simulink model "CollisionSim"  (R2015a)
settings: Solver=ode45  StartTime=0.0  StopTime=70  FixedStep=0.001  RelTol=1e-3
values from neighbouring files (symbols this model uses):
  Destination_Obs = [1000,0]    [CD.m]
  K_eta = 1    [CD.m]    (also in PathFollowCompScript.m = 0.21)
  lambda_0 = atan2(lambda_vec_0(2),lambda_vec_0(1))    [CD.m]    (also in PathFollowCompScript.m)
  V_obs_max = 20    [CD.m]
undefined symbols (not defined in the file): Initial_Head_Obs, Initial_Heading, Initial_Pos_Obs, Initial_Position
libraries: simulink x4, aerolibtransform2 x1
settings Model: CovSFcnEnable=off  Creator=marinho  LastModifiedBy=marinho
settings DebuggingCC: UnderspecifiedInitializationDetection=Classic  MergeDetectMultiDrivingBlocksExec=none  SolverPrmCheckMsg=warning

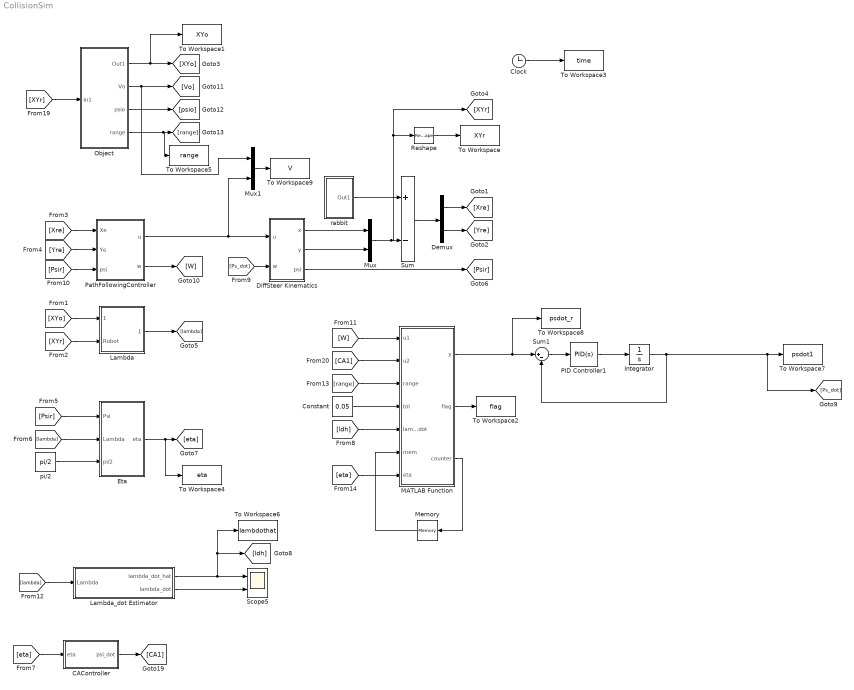
== system CollisionSim ==
  CAController : Subsystem
  Clock : Clock
  Constant : Constant  Value=0.05
  Demux : Demux  Outputs=2
  DiffSteer Kinematics : Subsystem  AncestorBlock=DiffSteer_model/DiffSteer Kinematics  mask{x0=[Initial_Position Initial_Heading], a=0.2, umax=32, wmax=5, dumax=inf, dwmax=inf}
      mask prompts: x0 "Initial pose [x, y, psi]"; a "Distance from traction wheels axis center to the point of interest [m]"; umax "Maximum linear velocity [m/s]"; wmax "Maximum angular velocity [rad/s]"; dumax "Maximum linear acceleration [m/s^2]"; dwmax "Maximum angular acceleration [rad/s^2]"
      mask help: Kinematics of the differential steered vehicle
      mask Help:
      | Kinematics of the differential steered vehicle (unicycle-like).
      | 
      | A differential steered (or differential wheeled) robot has two separately driven wheels placed on either side of its structure. Its orientation is changed by varying the relative velocities of its wheels.
      | In this model, robot position [x,y] is the position of the point of interest, which is located on a distance "a" from the center of the line that connects both traction wheels. If a = 0, this model is equal to the unicycle.
      | 
      | <b>Parameters:</b>
      | 
      | Initial pose: Vehicle initial position and orientation on absolute reference frame [x_0, y_0, psi_0]
      | Distance between traction wheels axis and point of interest (1x1): a [m]
      | Maximum Linear velocity (1x1):  Vehicle speed limit [m/s] (umax)
      | Maximum Angular velocity (1x1):  Vehicle turning velocity limit [rad/s] (wmax)
      | Maximum linear acceleration (1x1): Vehicle linear acceleration limit [m/s2] (dumax)
      | Maximum angular acceleration (1x1): Vehicle angular acceleration limit [rad/s2] (dwmax)
      | 
      | 
      | <b>Inputs:</b>
      | 
      | u (1x1): reference for linear velocity [m/s]
      | w (1x1): reference for angular velocity [rad/s]
      | 
      | <b>Outputs:</b>
      | 
      | x (1x1): x-coordinate in world frame [m]
      | y (1x1): y-coordinate in world frame [m]
      | psi (1x1): heading angle in world frame [rad]
      | 
      | <b>Notes:</b>
      | 
      | 1. If a = 0, this model is equal to the unicycle.
      | 
      | 2. This model does not take into account the robot dynamics. It considers that the actual robot velocity is exactly equal to the reference velocity (if it is bellow its limit).
      | 
      | For more information on the robot kinematics and dynamics, please refer to:
      | 
      | [1] MARTINS, F.N., CARELLI, R., SARCINELLI-FILHO, M. and BASTOS-FILHO, T.F.
      | Dynamic Modeling and Adaptive Dynamic Compensation for Unicycle-Like
      | Mobile Robots. 14th International Conference on Advanced Robotics -
      | ICAR 2009, Germany, June, 22-26, 2009.
      | 
      | [2] MARTINS, F.N., CELESTE, W.C., CARELLI, R., SARCINELLI-FILHO, M. and
      | BASTOS-FILHO, T.F. An Adaptive Dynamic Controller for Autonomous Mobile Robot
      | Trajectory Tracking. Control Engineering Practice, v. 16, p. 1354–1363, 2008.
      | doi: 10.1016/j.conengprac.2008.03.004
  Eta : Subsystem
  Integrator : Integrator  UpperSaturationLimit=0.5  LowerSaturationLimit=-0.5
  Lambda : Subsystem
  Lambda_dot Estimator : Subsystem
  MATLAB Function : MATLAB Function  TreatAsAtomicUnit=on
  Memory : Memory
  Mux : Mux  Inputs=2
  Mux1 : Mux  Inputs=2
  Object : Subsystem
  PID Controller1 : simulink/Continuous/PID Controller  Controller=PID  TimeDomain=Continuous-time  SampleTime=-1  IntegratorMethod=Forward Euler  FilterMethod=Forward Euler  Form=Parallel  UseFilter=on  ControllerParametersSource=internal  P=1  I=0  D=0.05  N=100  InitialConditionSource=internal  InitialConditionForIntegrator=0  InitialConditionForFilter=0  ExternalReset=none  LimitOutput=off  UpperSaturationLimit=0.1  LowerSaturationLimit=-0.1  LinearizeAsGain=on  AntiWindupMode=none  Kb=1  TrackingMode=off  Kt=1  PParamMin=[]  PParamMax=[]  IParamMin=[]  IParamMax=[]  DParamMin=[]  DParamMax=[]  NParamMin=[]  NParamMax=[]  KbParamMin=[]  KbParamMax=[]  KtParamMin=[]  KtParamMax=[]  POutMin=[]  POutMax=[]  IOutMin=[]  IOutMax=[]  DOutMin=[]  DOutMax=[]  NOutMin=[]  NOutMax=[]  KbOutMin=[]  KbOutMax=[]  KtOutMin=[]  KtOutMax=[]  IntegratorOutMin=[]  IntegratorOutMax=[]  FilterOutMin=[]  FilterOutMax=[]  SumOutMin=[]  SumOutMax=[]  SumI1OutMin=[]  SumI1OutMax=[]  SumI2OutMin=[]  SumI2OutMax=[]  SumI3OutMin=[]  SumI3OutMax=[]  SumDOutMin=[]  SumDOutMax=[]  SaturationOutMin=[]  SaturationOutMax=[]  IntegratorContinuousStateAttributes=''  IntegratorStateMustResolveToSignalObject=off  IntegratorRTWStateStorageClass=Auto  FilterContinuousStateAttributes=''  FilterStateMustResolveToSignalObject=off  FilterRTWStateStorageClass=Auto  DifferentiatorICPrevScaledInput=0  DifferentiatorOutMin=[]  DifferentiatorOutMax=[]
  PathFollowingController : Subsystem
  Reshape : Reshape
  Scope5 : Scope  NumInputPorts=2
      settings: YMin=-5~-5  YMax=5~5  SaveName=ScopeData10
  Sum : Sum  Inputs=+-
  Sum1 : Sum  Inputs=|+-
  To Workspace : ToWorkspace  VariableName=XYr  SampleTime=-1
  To Workspace1 : ToWorkspace  VariableName=XYo  SampleTime=-1
  To Workspace2 : ToWorkspace  VariableName=flag  SampleTime=-1
  To Workspace3 : ToWorkspace  VariableName=time  SampleTime=-1
  To Workspace4 : ToWorkspace  VariableName=eta  SampleTime=-1
  To Workspace5 : ToWorkspace  VariableName=range  SampleTime=-1
  To Workspace6 : ToWorkspace  VariableName=lambdothat  SampleTime=-1
  To Workspace7 : ToWorkspace  VariableName=psdot1  SampleTime=-1
  To Workspace8 : ToWorkspace  VariableName=psdot_r  SampleTime=-1
  To Workspace9 : ToWorkspace  VariableName=V  SampleTime=-1
  "pi/2 " : Constant  Value=pi/2  VectorParams1D=off  SampleTime=-1
  rabbit : Subsystem
  wires:
  DiffSteer Kinematics/1(x) -> Mux/1
  DiffSteer Kinematics/2(y) -> Mux/2
  Mux/1 -> Sum/2, [XYr], Reshape/1
  rabbit/1(Out1) -> Sum/1
  Sum/1 -> Demux/1
  Demux/2 -> [Yre]
  Demux/1 -> [Xre]
  Reshape/1 -> To Workspace/1
  DiffSteer Kinematics/3(psi) -> [Psir]
  [Xre] -> PathFollowingController/1(Xe)
  [Yre] -> PathFollowingController/2(Ye)
  [Psir] -> PathFollowingController/3(psi)
  PathFollowingController/1(u) -> Mux1/2, DiffSteer Kinematics/1(u)
  [W] -> MATLAB Function/1(u1)
  Clock/1 -> To Workspace3/1
  PathFollowingController/2(w) -> [W]
  [lambda] -> Lambda_dot Estimator/1(Lambda)
  Object/2(Vo) -> Mux1/1, [Vo]
  Object/3(psio) -> [psio]
  [XYr] -> Object/1(In1)
  MATLAB Function/2(flag) -> To Workspace2/1
  Lambda_dot Estimator/1(lambda_dot_hat) -> [ldh], To Workspace6/1, Scope5/1
  Lambda_dot Estimator/2(lambda_dot) -> Scope5/2
  Object/4(range) -> To Workspace5/1, [range]
  [range] -> MATLAB Function/3(range)
  MATLAB Function/3(counter) -> Memory/1
  Memory/1 -> MATLAB Function/6(mem)
  Constant/1 -> MATLAB Function/4(tol)
  [eta] -> MATLAB Function/7(eta)
  [Ps_dot] -> DiffSteer Kinematics/2(w)
  Object/1(Out1) -> To Workspace1/1, [XYo]
  [XYo] -> Lambda/1(Object)
  [XYr] -> Lambda/2(Robot)
  Lambda/1(Lambda) -> [lambda]
  Eta/1(eta) -> To Workspace4/1, [eta]
  [Psir] -> Eta/1(Psi)
  [lambda] -> Eta/2(Lambda)
  "pi/2 "/1 -> Eta/3(pi/2)
  [ldh] -> MATLAB Function/5(lambda_dot)
  [eta] -> CAController/1(eta)
  CAController/1(psi_dot) -> [CA1]
  Sum1/1 -> PID Controller1/1
  PID Controller1/1 -> Integrator/1
  MATLAB Function/1(y) -> To Workspace8/1, Sum1/1
  Integrator/1 -> [Ps_dot], To Workspace7/1, Sum1/2
  Mux1/1 -> To Workspace9/1
  [CA1] -> MATLAB Function/2(u2)

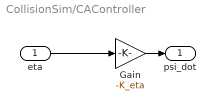
== system CollisionSim/CAController ==
  eta : Inport
  Gain : Gain  Gain=-K_eta
  psi_dot : Outport
  wires:
  Gain/1 -> psi_dot/1
  eta/1 -> Gain/1

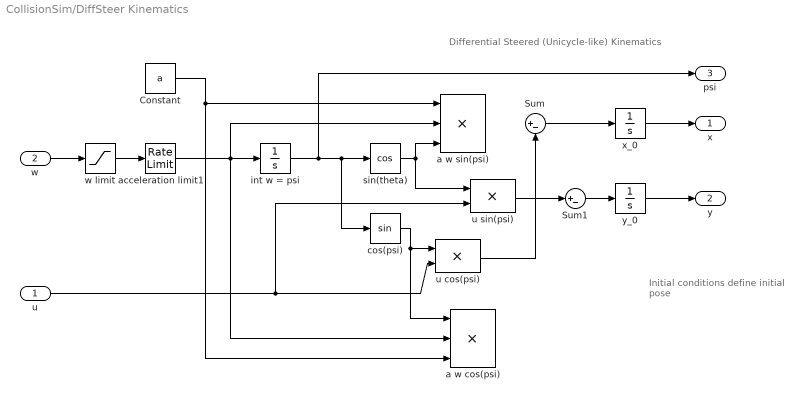
== system CollisionSim/DiffSteer Kinematics ==
  note: Differential Steered (Unicycle-like) Kinematics
  note: Initial conditions define
      | initial pose
  u : Inport
  w : Inport  Port=2
  Constant : Constant  Value=a
  Sum : Sum  Inputs=|+-  SaturateOnIntegerOverflow=on
  Sum1 : Sum  Inputs=|+-  SaturateOnIntegerOverflow=on
  a w cos(psi) : Product  Inputs=3  SaturateOnIntegerOverflow=on  OutDataTypeStr=Inherit: Same as first input
  a w sin(psi) : Product  Inputs=3  SaturateOnIntegerOverflow=on  OutDataTypeStr=Inherit: Same as first input
  acceleration limit1 : RateLimiter  RisingSlewLimit=dwmax  FallingSlewLimit=-dwmax  SampleTimeMode=inherited
  cos(psi) : Trigonometry
  int w = psi : Integrator  InitialCondition=x0(3)
  sin(theta) : Trigonometry  Operator=cos
  u cos(psi) : Product  SaturateOnIntegerOverflow=on  OutDataTypeStr=Inherit: Same as first input
  u sin(psi) : Product  SaturateOnIntegerOverflow=on  OutDataTypeStr=Inherit: Same as first input
  w limit : Saturate  UpperLimit=wmax  LowerLimit=-wmax
  x_0 : Integrator  InitialCondition=x0(1)
  y_0 : Integrator  InitialCondition=x0(2)
  x : Outport
  y : Outport  Port=2
  psi : Outport  Port=3
  wires:
  y_0/1 -> y/1
  Sum1/1 -> y_0/1
  u/1 -> u cos(psi)/2, u sin(psi)/2
  int w = psi/1 -> cos(psi)/1, sin(theta)/1, psi/1
  sin(theta)/1 -> u sin(psi)/1, a w sin(psi)/3
  Sum/1 -> x_0/1
  x_0/1 -> x/1
  Constant/1 -> a w cos(psi)/3, a w sin(psi)/1
  acceleration limit1/1 -> a w cos(psi)/2, int w = psi/1, a w sin(psi)/2
  cos(psi)/1 -> a w cos(psi)/1, u cos(psi)/1
  u sin(psi)/1 -> Sum1/1
  u cos(psi)/1 -> Sum/2
  w/1 -> w limit/1
  w limit/1 -> acceleration limit1/1

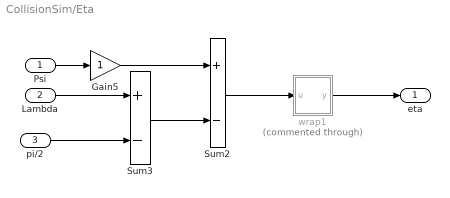
== system CollisionSim/Eta ==
  Psi : Inport
  Lambda : Inport  Port=2
  pi/2 : Inport  Port=3
  Gain5 : Gain
  Sum2 : Sum  Inputs=+-
  Sum3 : Sum  Inputs=+-
  wrap1 : MATLAB Function  Commented=through  TreatAsAtomicUnit=on
  eta : Outport
  wires:
  wrap1/1(y) -> eta/1
  Psi/1 -> Gain5/1
  Lambda/1 -> Sum3/1
  Sum3/1 -> Sum2/2
  pi/2/1 -> Sum3/2
  Sum2/1 -> wrap1/1(u)
  Gain5/1 -> Sum2/1

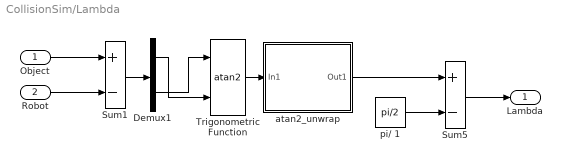
== system CollisionSim/Lambda ==
  Object : Inport
  Robot : Inport  Port=2
  Demux1 : Demux  Outputs=2
  Sum1 : Sum  Inputs=+-
  Sum5 : Sum  Inputs=+-
  Trigonometric Function : Trigonometry  Operator=atan2
  atan2_unwrap : Subsystem
  pi/ 1 : Constant  Value=pi/2  VectorParams1D=off  SampleTime=-1
  Lambda : Outport
  wires:
  Trigonometric Function/1 -> atan2_unwrap/1(In1)
  Demux1/2 -> Trigonometric Function/1
  pi/ 1/1 -> Sum5/2
  Sum5/1 -> Lambda/1
  atan2_unwrap/1(Out1) -> Sum5/1
  Sum1/1 -> Demux1/1
  Demux1/1 -> Trigonometric Function/2
  Object/1 -> Sum1/1
  Robot/1 -> Sum1/2

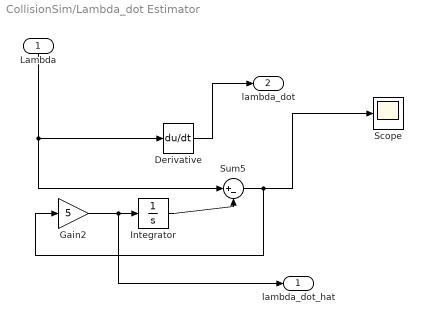
== system CollisionSim/Lambda_dot Estimator ==
  Lambda : Inport
  Derivative : Derivative
  Gain2 : Gain  Gain=5
  Integrator : Integrator
  Scope : Scope
  Sum5 : Sum  Inputs=|+-
  lambda_dot_hat : Outport
  lambda_dot : Outport  Port=2
  wires:
  Sum5/1 -> Scope/1, Gain2/1
  Gain2/1 -> lambda_dot_hat/1, Integrator/1
  Integrator/1 -> Sum5/2
  Lambda/1 -> Derivative/1, Sum5/1
  Derivative/1 -> lambda_dot/1

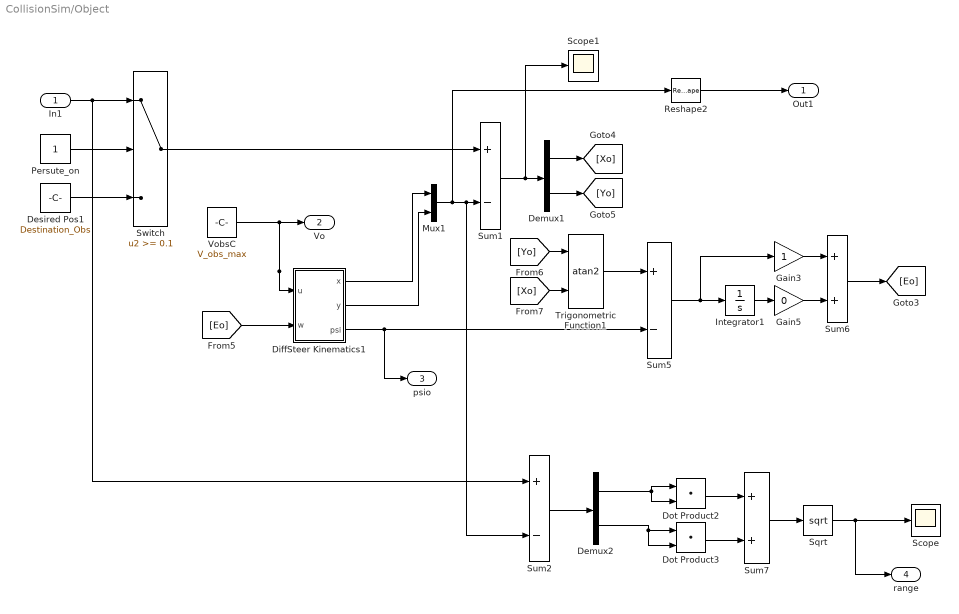
== system CollisionSim/Object ==
  In1 : Inport
  Demux1 : Demux  Outputs=2
  Demux2 : Demux  Outputs=2
  Desired Pos1 : Constant  Value=Destination_Obs  VectorParams1D=off  SampleTime=0.02
  DiffSteer Kinematics1 : Subsystem  AncestorBlock=DiffSteer_model/DiffSteer Kinematics  mask{x0=[Initial_Pos_Obs Initial_Head_Obs], a=0.2, umax=40, wmax=5, dumax=inf, dwmax=inf}
      mask prompts: x0 "Initial pose [x, y, psi]"; a "Distance from traction wheels axis center to the point of interest [m]"; umax "Maximum linear velocity [m/s]"; wmax "Maximum angular velocity [rad/s]"; dumax "Maximum linear acceleration [m/s^2]"; dwmax "Maximum angular acceleration [rad/s^2]"
      mask help: Kinematics of the differential steered vehicle
      mask Help:
      | Kinematics of the differential steered vehicle (unicycle-like).
      | 
      | A differential steered (or differential wheeled) robot has two separately driven wheels placed on either side of its structure. Its orientation is changed by varying the relative velocities of its wheels.
      | In this model, robot position [x,y] is the position of the point of interest, which is located on a distance "a" from the center of the line that connects both traction wheels. If a = 0, this model is equal to the unicycle.
      | 
      | <b>Parameters:</b>
      | 
      | Initial pose: Vehicle initial position and orientation on absolute reference frame [x_0, y_0, psi_0]
      | Distance between traction wheels axis and point of interest (1x1): a [m]
      | Maximum Linear velocity (1x1):  Vehicle speed limit [m/s] (umax)
      | Maximum Angular velocity (1x1):  Vehicle turning velocity limit [rad/s] (wmax)
      | Maximum linear acceleration (1x1): Vehicle linear acceleration limit [m/s2] (dumax)
      | Maximum angular acceleration (1x1): Vehicle angular acceleration limit [rad/s2] (dwmax)
      | 
      | 
      | <b>Inputs:</b>
      | 
      | u (1x1): reference for linear velocity [m/s]
      | w (1x1): reference for angular velocity [rad/s]
      | 
      | <b>Outputs:</b>
      | 
      | x (1x1): x-coordinate in world frame [m]
      | y (1x1): y-coordinate in world frame [m]
      | psi (1x1): heading angle in world frame [rad]
      | 
      | <b>Notes:</b>
      | 
      | 1. If a = 0, this model is equal to the unicycle.
      | 
      | 2. This model does not take into account the robot dynamics. It considers that the actual robot velocity is exactly equal to the reference velocity (if it is bellow its limit).
      | 
      | For more information on the robot kinematics and dynamics, please refer to:
      | 
      | [1] MARTINS, F.N., CARELLI, R., SARCINELLI-FILHO, M. and BASTOS-FILHO, T.F.
      | Dynamic Modeling and Adaptive Dynamic Compensation for Unicycle-Like
      | Mobile Robots. 14th International Conference on Advanced Robotics -
      | ICAR 2009, Germany, June, 22-26, 2009.
      | 
      | [2] MARTINS, F.N., CELESTE, W.C., CARELLI, R., SARCINELLI-FILHO, M. and
      | BASTOS-FILHO, T.F. An Adaptive Dynamic Controller for Autonomous Mobile Robot
      | Trajectory Tracking. Control Engineering Practice, v. 16, p. 1354–1363, 2008.
      | doi: 10.1016/j.conengprac.2008.03.004
  Dot Product2 : DotProduct  InputSameDT=on  OutDataTypeStr=Inherit: Inherit via internal rule
  Dot Product3 : DotProduct  InputSameDT=on  OutDataTypeStr=Inherit: Inherit via internal rule
  Gain3 : Gain
  Gain5 : Gain  Gain=0
  Integrator1 : Integrator
  Mux1 : Mux  Inputs=2
  Persute_on : Constant  VectorParams1D=off  SampleTime=0.02
  Reshape2 : Reshape
  Scope : Scope
      settings: SaveName=ScopeData8
  Scope1 : Scope
      settings: SaveName=ScopeData7
  Sqrt : Sqrt  SaturateOnIntegerOverflow=on
  Sum1 : Sum  Inputs=+-
  Sum2 : Sum  Inputs=+-
  Sum5 : Sum  Inputs=+-
  Sum6 : Sum
  Sum7 : Sum
  Switch : Switch  Threshold=0.1
  Trigonometric Function1 : Trigonometry  Operator=atan2
  VobsC : Constant  Value=V_obs_max  VectorParams1D=off  SampleTime=0.02
  Out1 : Outport
  Vo : Outport  Port=2
  psio : Outport  Port=3
  range : Outport  Port=4
  wires:
  Sum6/1 -> [Eo]
  [Eo] -> DiffSteer Kinematics1/2(w)
  Dot Product2/1 -> Sum7/1
  Sum7/1 -> Sqrt/1
  Demux1/2 -> [Yo]
  [Yo] -> Trigonometric Function1/1
  Demux2/1 -> Dot Product2/1, Dot Product2/2
  Demux1/1 -> [Xo]
  [Xo] -> Trigonometric Function1/2
  Mux1/1 -> Reshape2/1, Sum2/2, Sum1/2
  Dot Product3/1 -> Sum7/2
  Demux2/2 -> Dot Product3/2, Dot Product3/1
  Sum1/1 -> Scope1/1, Demux1/1
  DiffSteer Kinematics1/2(y) -> Mux1/2
  DiffSteer Kinematics1/1(x) -> Mux1/1
  Sum5/1 -> Gain3/1, Integrator1/1
  Trigonometric Function1/1 -> Sum5/1
  Gain5/1 -> Sum6/2
  Gain3/1 -> Sum6/1
  DiffSteer Kinematics1/3(psi) -> psio/1, Sum5/2
  Integrator1/1 -> Gain5/1
  Reshape2/1 -> Out1/1
  VobsC/1 -> Vo/1, DiffSteer Kinematics1/1(u)
  Sqrt/1 -> range/1, Scope/1
  Persute_on/1 -> Switch/2
  In1/1 -> Sum2/1, Switch/1
  Desired Pos1/1 -> Switch/3
  Switch/1 -> Sum1/1
  Sum2/1 -> Demux2/1

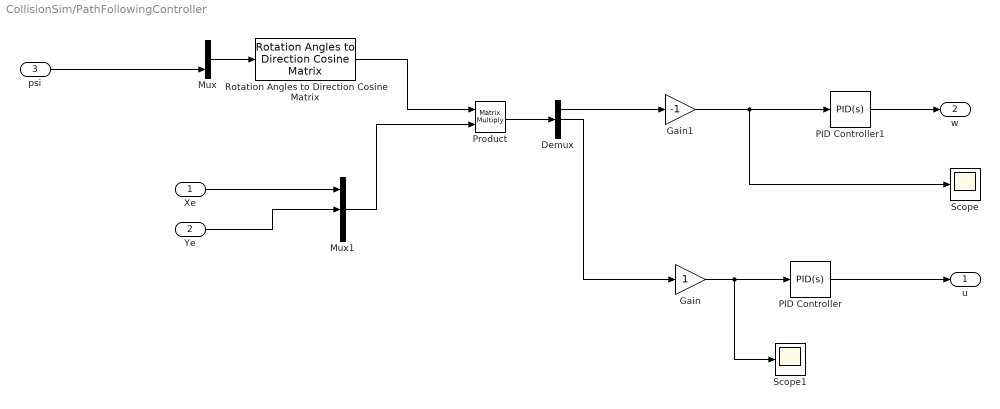
== system CollisionSim/PathFollowingController ==
  Xe : Inport
  Ye : Inport  Port=2
  psi : Inport  Port=3
  Demux : Demux  Outputs=3
  Gain : Gain
  Gain1 : Gain  Gain=-1
  Mux : Mux  Inputs=3
  Mux1 : Mux  Inputs=3
  PID Controller : simulink/Continuous/PID Controller  Controller=PID  TimeDomain=Continuous-time  SampleTime=-1  IntegratorMethod=Forward Euler  FilterMethod=Forward Euler  Form=Parallel  UseFilter=on  ControllerParametersSource=internal  P=1.5  I=0  D=0  N=100  InitialConditionSource=internal  InitialConditionForIntegrator=0  InitialConditionForFilter=0  ExternalReset=none  LimitOutput=on  UpperSaturationLimit=24  LowerSaturationLimit=14  LinearizeAsGain=on  AntiWindupMode=none  Kb=1  TrackingMode=off  Kt=1  PParamMin=[]  PParamMax=[]  IParamMin=[]  IParamMax=[]  DParamMin=[]  DParamMax=[]  NParamMin=[]  NParamMax=[]  KbParamMin=[]  KbParamMax=[]  KtParamMin=[]  KtParamMax=[]  POutMin=[]  POutMax=[]  IOutMin=[]  IOutMax=[]  DOutMin=[]  DOutMax=[]  NOutMin=[]  NOutMax=[]  KbOutMin=[]  KbOutMax=[]  KtOutMin=[]  KtOutMax=[]  IntegratorOutMin=[]  IntegratorOutMax=[]  FilterOutMin=[]  FilterOutMax=[]  SumOutMin=[]  SumOutMax=[]  SumI1OutMin=[]  SumI1OutMax=[]  SumI2OutMin=[]  SumI2OutMax=[]  SumI3OutMin=[]  SumI3OutMax=[]  SumDOutMin=[]  SumDOutMax=[]  SaturationOutMin=[]  SaturationOutMax=[]  IntegratorContinuousStateAttributes=''  IntegratorStateMustResolveToSignalObject=off  IntegratorRTWStateStorageClass=Auto  FilterContinuousStateAttributes=''  FilterStateMustResolveToSignalObject=off  FilterRTWStateStorageClass=Auto  DifferentiatorICPrevScaledInput=0  DifferentiatorOutMin=[]  DifferentiatorOutMax=[]
  PID Controller1 : simulink/Continuous/PID Controller  Controller=PID  TimeDomain=Continuous-time  SampleTime=-1  IntegratorMethod=Forward Euler  FilterMethod=Forward Euler  Form=Parallel  UseFilter=on  ControllerParametersSource=internal  P=0.01  I=0  D=0.01  N=100  InitialConditionSource=internal  InitialConditionForIntegrator=0  InitialConditionForFilter=0  ExternalReset=none  LimitOutput=on  UpperSaturationLimit=0.2  LowerSaturationLimit=-0.2  LinearizeAsGain=on  AntiWindupMode=none  Kb=1  TrackingMode=off  Kt=1  PParamMin=[]  PParamMax=[]  IParamMin=[]  IParamMax=[]  DParamMin=[]  DParamMax=[]  NParamMin=[]  NParamMax=[]  KbParamMin=[]  KbParamMax=[]  KtParamMin=[]  KtParamMax=[]  POutMin=[]  POutMax=[]  IOutMin=[]  IOutMax=[]  DOutMin=[]  DOutMax=[]  NOutMin=[]  NOutMax=[]  KbOutMin=[]  KbOutMax=[]  KtOutMin=[]  KtOutMax=[]  IntegratorOutMin=[]  IntegratorOutMax=[]  FilterOutMin=[]  FilterOutMax=[]  SumOutMin=[]  SumOutMax=[]  SumI1OutMin=[]  SumI1OutMax=[]  SumI2OutMin=[]  SumI2OutMax=[]  SumI3OutMin=[]  SumI3OutMax=[]  SumDOutMin=[]  SumDOutMax=[]  SaturationOutMin=[]  SaturationOutMax=[]  IntegratorContinuousStateAttributes=''  IntegratorStateMustResolveToSignalObject=off  IntegratorRTWStateStorageClass=Auto  FilterContinuousStateAttributes=''  FilterStateMustResolveToSignalObject=off  FilterRTWStateStorageClass=Auto  DifferentiatorICPrevScaledInput=0  DifferentiatorOutMin=[]  DifferentiatorOutMax=[]
  Product : Product  Multiplication=Matrix(*)
  Rotation Angles to Direction Cosine Matrix : aerolibtransform2/Rotation Angles to Direction Cosine Matrix  rotationOrder=XYZ
  Scope : Scope
      settings: SaveName=ScopeData5
  Scope1 : Scope
      settings: YMin=8750  YMax=12500  SaveName=ScopeData6
  u : Outport
  w : Outport  Port=2
  wires:
  psi/1 -> Mux/3
  Mux/1 -> Rotation Angles to Direction Cosine Matrix/1
  Rotation Angles to Direction Cosine Matrix/1 -> Product/1
  Mux1/1 -> Product/2
  Product/1 -> Demux/1
  Demux/1 -> Gain1/1
  Demux/2 -> Gain/1
  Gain/1 -> Scope1/1, PID Controller/1
  Gain1/1 -> Scope/1, PID Controller1/1
  PID Controller1/1 -> w/1
  Xe/1 -> Mux1/1
  Ye/1 -> Mux1/2
  PID Controller/1 -> u/1

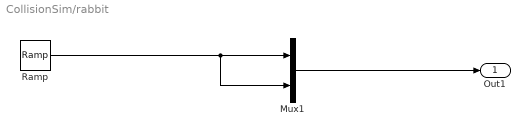
== system CollisionSim/rabbit ==
  Mux1 : Mux  Inputs=2
  Ramp : simulink/Sources/Ramp  slope=20/sqrt(2)  start=0  X0=100
  Out1 : Outport
  wires:
  Ramp/1 -> Mux1/2, Mux1/1
  Mux1/1 -> Out1/1

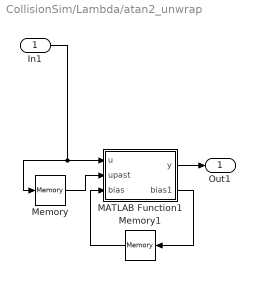
== system CollisionSim/Lambda/atan2_unwrap ==
  In1 : Inport
  MATLAB Function1 : MATLAB Function  TreatAsAtomicUnit=on
  Memory : Memory  X0=lambda_0
  Memory1 : Memory
  Out1 : Outport
  wires:
  In1/1 -> Memory/1, MATLAB Function1/1(u)
  Memory/1 -> MATLAB Function1/2(upast)
  MATLAB Function1/1(y) -> Out1/1
  MATLAB Function1/2(bias1) -> Memory1/1
  Memory1/1 -> MATLAB Function1/3(bias)

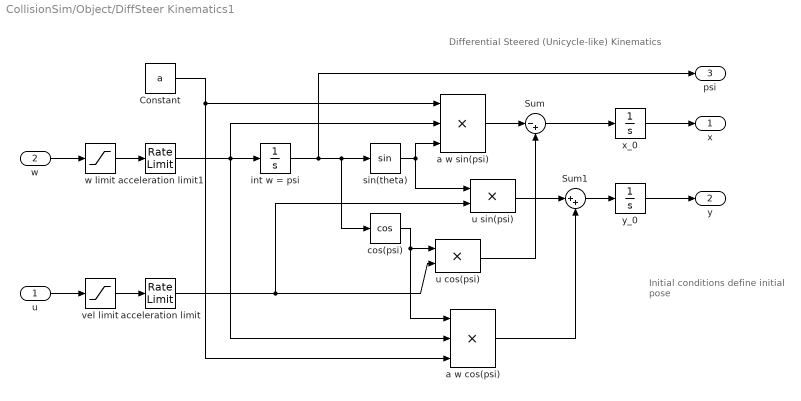
== system CollisionSim/Object/DiffSteer Kinematics1 ==
  note: Differential Steered (Unicycle-like) Kinematics
  note: Initial conditions define
      | initial pose
  u : Inport
  w : Inport  Port=2
  Constant : Constant  Value=a
  Sum : Sum  Inputs=|-+  SaturateOnIntegerOverflow=on
  Sum1 : Sum  Inputs=|++  SaturateOnIntegerOverflow=on
  a w cos(psi) : Product  Inputs=3  SaturateOnIntegerOverflow=on  OutDataTypeStr=Inherit: Same as first input
  a w sin(psi) : Product  Inputs=3  SaturateOnIntegerOverflow=on  OutDataTypeStr=Inherit: Same as first input
  acceleration limit : RateLimiter  RisingSlewLimit=dumax  FallingSlewLimit=-dumax  SampleTimeMode=inherited
  acceleration limit1 : RateLimiter  RisingSlewLimit=dwmax  FallingSlewLimit=-dwmax  SampleTimeMode=inherited
  cos(psi) : Trigonometry  Operator=cos
  int w = psi : Integrator  InitialCondition=x0(3)
  sin(theta) : Trigonometry
  u cos(psi) : Product  SaturateOnIntegerOverflow=on  OutDataTypeStr=Inherit: Same as first input
  u sin(psi) : Product  SaturateOnIntegerOverflow=on  OutDataTypeStr=Inherit: Same as first input
  vel limit : Saturate  UpperLimit=umax  LowerLimit=-umax
  w limit : Saturate  UpperLimit=wmax  LowerLimit=-wmax
  x_0 : Integrator  InitialCondition=x0(1)
  y_0 : Integrator  InitialCondition=x0(2)
  x : Outport
  y : Outport  Port=2
  psi : Outport  Port=3
  wires:
  y_0/1 -> y/1
  Sum1/1 -> y_0/1
  a w sin(psi)/1 -> Sum/1
  acceleration limit/1 -> u cos(psi)/2, u sin(psi)/2
  u cos(psi)/1 -> Sum/2
  vel limit/1 -> acceleration limit/1
  int w = psi/1 -> cos(psi)/1, sin(theta)/1, psi/1
  w/1 -> w limit/1
  a w cos(psi)/1 -> Sum1/2
  sin(theta)/1 -> u sin(psi)/1, a w sin(psi)/3
  Sum/1 -> x_0/1
  u/1 -> vel limit/1
  x_0/1 -> x/1
  Constant/1 -> a w cos(psi)/3, a w sin(psi)/1
  w limit/1 -> acceleration limit1/1
  acceleration limit1/1 -> int w = psi/1, a w sin(psi)/2, a w cos(psi)/2
  cos(psi)/1 -> a w cos(psi)/1, u cos(psi)/1
  u sin(psi)/1 -> Sum1/1

== matlab function CollisionSim/Lambda/atan2_unwrap/MATLAB Function1 ==
  data: u input; y output; upast input; bias input; bias1 output
function [y, bias1] = fcn(u,upast,bias)
newbias = 0;
if u-upast > 3*pi/2
    newbias = -4*pi/2;
end
if u-upast < -3*pi/2
   newbias = +4*pi/2;
end
bias1 = bias + newbias;
y = u+bias1;

== matlab function CollisionSim/MATLAB Function ==
  data: u1 input; y output; u2 input; range input; flag output; tol input; lambda_dot input; mem input; counter output; eta input
function [y,flag,counter] = fcn(u1,u2,range,tol, lambda_dot,mem,eta)
y=u1;
flag = 0;
if (range <= 400)
    if ((abs(lambda_dot) < tol) && eta > 0)
        mem = 420;
        y= u1 + u2;
        flag = 1;
    end
    if mem > 0
        y=u1 + u2;
        flag = 1;
    end
else
    y = u1;
    flag = 0;
end
counter = mem -1;

== matlab function CollisionSim/Eta/wrap1 ==
  data: u input; y output
function y = fcn(u)
%#codegen

u2 = mod(u+pi/2,pi/2);

y = u2;
